simulink model "if_else_subsystem_ejemplo"  (Simulink 7.1)
settings: Solver=ode45  StartTime=0.0  StopTime=10.0  MaxStep=0.05  RelTol=1e-3
settings Model: Creator=Usuario  LastModifiedBy=Usuario

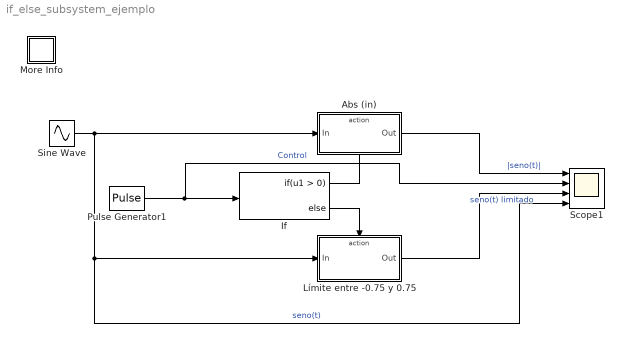
== system if_else_subsystem_ejemplo ==
  Abs (in) : Subsystem  TreatAsAtomicUnit=on
  If : If
  Límite entre -0.75 y 0.75 : Subsystem  TreatAsAtomicUnit=on
  More Info : Subsystem
      settings: OpenFcn=showdemo(bdroot(gcb))
      mask Display: disp('?')
  Pulse Generator1 : DiscretePulseGenerator  PulseType=Time based  Period=5  PulseWidth=50
      settings: AttributesFormatString=Period: %<period>\nDuty cycle: %<pulsewidth>%
  Scope1 : Scope  NumInputPorts=4
      settings: StartFcn=open_system(gcbh)  TickLabels=on  TimeRange=10  YMin=-1.6~-0.1~-1.5~-5  YMax=3.6~1.1~3.5~5  DataFormat=Structure
  Sine Wave : Sin  SampleTime=0
  wires:
  Sine Wave/1 -> Abs (in)/1(In), Límite entre -0.75 y 0.75/1(In), Scope1/4  "seno(t)"
  Pulse Generator1/1 -> If/1, Scope1/2  "Control"
  If/2 -> Límite entre -0.75 y 0.75/Action
  If/1 -> Abs (in)/Action
  Abs (in)/1(Out) -> Scope1/1  "|seno(t)|"
  Límite entre -0.75 y 0.75/1(Out) -> Scope1/3  "seno(t) limitado"

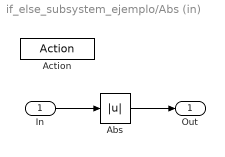
== system if_else_subsystem_ejemplo/Abs (in) ==
  In : Inport  OutDataType=sfix(16)  OutScaling=2^0
  Action : ActionPort  InitializeStates=reset  ActionType=then
  Abs : Abs  SaturateOnIntegerOverflow=on
  Out : Outport  OutDataType=sfix(16)  OutScaling=2^0  OutputWhenDisabled=reset  InitialOutput=0
  wires:
  In/1 -> Abs/1
  Abs/1 -> Out/1

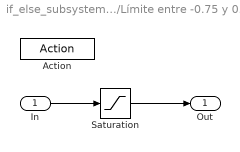
== system if_else_subsystem_ejemplo/Límite entre -0.75 y 0.75 ==
  In : Inport  OutDataType=sfix(16)  OutScaling=2^0
  Action : ActionPort  ActionType=else
  Saturation : Saturate  UpperLimit=0.75  LowerLimit=-0.75
  Out : Outport  OutDataType=sfix(16)  OutScaling=2^0
  wires:
  Saturation/1 -> Out/1
  In/1 -> Saturation/1

== system if_else_subsystem_ejemplo/More Info ==
